simulink model "uz_pmsm_model_nonlinear"  (R2024b)
settings: Solver=FixedStepDiscrete  StartTime=0.0  StopTime=0.5  RelTol=1e-3
PreLoadFcn:
  | uz_pmsm_model_nonlinear_init_parameter
values from neighbouring files (symbols this model uses):
  ad1 = ad_1(1)    [LUT_approx_methode2a.m]    (also in LUT_approx_methode2a_clean.m = ad_self(1); LUT_approx_methode_2a_FEM.m; fitting_parameter.mat = 0.03048394862; fitting_parameter_48V_SynRM.mat = 0.0218446789236)
  ad2 = ad_1(2)    [LUT_approx_methode2a.m]    (also in LUT_approx_methode2a_clean.m = ad_self(2); LUT_approx_methode_2a_FEM.m; fitting_parameter.mat = 0.0402440194669; fitting_parameter_48V_SynRM.mat = 0.015691946268)
  ad3 = ad_1(3)    [LUT_approx_methode2a.m]    (also in LUT_approx_methode2a_clean.m = ad_self(3); LUT_approx_methode_2a_FEM.m; fitting_parameter.mat = -16.4812001193; fitting_parameter_48V_SynRM.mat = 2.77465564774)
  ad4 = ad_3_6(1)    [LUT_approx_methode2a.m]    (also in LUT_approx_methode2a_clean.m = ad_4_6(1); LUT_approx_methode_2a_FEM.m; fitting_parameter.mat = 1.2964378241; fitting_parameter_48V_SynRM.mat = 0.0214529395212)
  ad5 = ad_3_6(2)    [LUT_approx_methode2a.m]    (also in LUT_approx_methode2a_clean.m = ad_4_6(2); LUT_approx_methode_2a_FEM.m; fitting_parameter.mat = 0.000618316734858; fitting_parameter_48V_SynRM.mat = 0.0128514742508)
  ad6 = ad_3_6(3)    [LUT_approx_methode2a.m]    (also in LUT_approx_methode2a_clean.m = ad_4_6(3); LUT_approx_methode_2a_FEM.m; fitting_parameter.mat = -12.2755860444; fitting_parameter_48V_SynRM.mat = 2.54408267654)
  aq1 = aq_1(1)    [LUT_approx_methode2a.m]    (also in LUT_approx_methode2a_clean.m = aq_self(1); LUT_approx_methode_2a_FEM.m; fitting_parameter.mat = 0.0048166705291; fitting_parameter_48V_SynRM.mat = 0.00205546577039)
  aq2 = aq_1(2)    [LUT_approx_methode2a.m]    (also in LUT_approx_methode2a_clean.m = aq_self(2); LUT_approx_methode_2a_FEM.m; fitting_parameter.mat = 0.171595255564; fitting_parameter_48V_SynRM.mat = 0.0602932843871)
  aq3 = aq_1(3)    [LUT_approx_methode2a.m]    (also in LUT_approx_methode2a_clean.m = aq_self(3); LUT_approx_methode_2a_FEM.m; fitting_parameter.mat = 0.000926293864031; fitting_parameter_48V_SynRM.mat = 4.42738872822e-05)
  aq4 = aq_3_6(1)    [LUT_approx_methode2a.m]    (also in LUT_approx_methode2a_clean.m = aq_4_6(1); LUT_approx_methode_2a_FEM.m; fitting_parameter.mat = 0.00500187099075; fitting_parameter_48V_SynRM.mat = 0.000698420875152)
  aq5 = aq_3_6(2)    [LUT_approx_methode2a.m]    (also in LUT_approx_methode2a_clean.m = aq_4_6(2); LUT_approx_methode_2a_FEM.m; fitting_parameter.mat = 0.17052123489; fitting_parameter_48V_SynRM.mat = 0.0493122483219)
  aq6 = aq_3_6(3)    [LUT_approx_methode2a.m]    (also in LUT_approx_methode2a_clean.m = aq_4_6(3); LUT_approx_methode_2a_FEM.m; fitting_parameter.mat = 0.00091860845; fitting_parameter_48V_SynRM.mat = 4.14644316065e-05)
  Fid1_Giq1 = ((1/2).*(aq3-aq6).*((q_current_set).^2))+((aq1./aq2).*log(cosh(aq2.*q_current_set)))-((aq4/aq5).*log(cosh(aq5.*q_current_set)))    [LUT_approx_methode2a.m]    (also in LUT_approx_methode2a_clean.m; LUT_approx_methode_2a_FEM.m = (1/2).*(aq3-aq6).*((q_current_set).^2)+((aq1./aq2).*log(cosh; fitting_parameter.mat = -0.00135679401385; fitting_parameter_48V_SynRM.mat = 0.221350145237)
  Fid2_Giq2 = ((ad1./ad2).*(log(cosh(ad2.*(d_current_set-ad3))))) - ((ad4./ad5).*(log(cosh(ad5.*(d_current_set-ad6)))))    [LUT_approx_methode2a.m]    (also in LUT_approx_methode2a_clean.m; LUT_approx_methode_2a_FEM.m = ((ad1./ad2).*(log(cosh(ad2.*(d_current_set-ad3))))) - (((ad1; fitting_parameter.mat = 0.0788137932988; fitting_parameter_48V_SynRM.mat = 0.221214979406)
  friction_coefficient = 0.001    [uz_pmsm_model_init_parameter.m]    (also in uz_pmsm_model_init_parameter_clean.m)
  inertia = 0.000084    (= 8.4e-05)    [uz_pmsm_model_init_parameter.m]    (also in uz_pmsm_model_init_parameter_clean.m)
  k_i_d = R_1/(2*tau_sum)    (= 1875)    [uz_pmsm_model_init_parameter.m]    (also in uz_pmsm_model_init_parameter_clean.m)
  k_p_d = L_d/(2*tau_sum)    (= 2.8125)    [uz_pmsm_model_init_parameter.m]    (also in uz_pmsm_model_init_parameter_clean.m)
  k_p_q = L_q/(2*tau_sum)    (= 12.5)    [uz_pmsm_model_init_parameter.m]    (also in uz_pmsm_model_init_parameter_clean.m)
  L_d = 0.00045    [uz_pmsm_model_init_parameter.m]    (also in uz_pmsm_model_init_parameter_clean.m)
  L_q = 0.002    [uz_pmsm_model_init_parameter.m]    (also in uz_pmsm_model_init_parameter_clean.m)
  polepair = 4    [uz_pmsm_model_init_parameter.m]    (also in uz_pmsm_model_init_parameter_clean.m)
  psi_pm = 0.0194    [uz_pmsm_model_init_parameter.m]    (also in uz_pmsm_model_init_parameter_clean.m)
  R_1 = 0.3    [uz_pmsm_model_init_parameter.m]    (also in uz_pmsm_model_init_parameter_clean.m)
  setpoint_step = 4.0    (= 4)    [compare_simulation_to_measurement.m]    (also in export_csv.m = 10; iae_von_cil_measurements.m = 8; uz_pmsm_model_init_parameter.m = 10; uz_pmsm_model_init_parameter_clean.m = 10)
  simulate_mechanical = true    [compare_simulation_to_measurement.m]    (also in export_csv.m = false; uz_pmsm_model_init_parameter.m = false; uz_pmsm_model_init_parameter_clean.m = false)
  simulate_open_loop = true    [compare_simulation_to_measurement.m]    (also in export_csv.m; uz_pmsm_model_init_parameter.m = false; uz_pmsm_model_init_parameter_clean.m = false)
  static_friction_torque = 0.01    [uz_pmsm_model_init_parameter.m]    (also in uz_pmsm_model_init_parameter_clean.m)
  ts = logs{k}.Values    [export_csv.m]    (also in uz_pmsm_model_init_parameter.m = 2e-06; uz_pmsm_model_init_parameter_clean.m = 2e-06)
  ts_regler = 1/25e3    (= 4e-05)    [uz_pmsm_model_init_parameter.m]    (also in uz_pmsm_model_init_parameter_clean.m)
undefined symbols (not defined in the file or in its folder): simulate_nonlinear
libraries: slpidlib x2
settings Model: DataTypeOverride=Off  Creator=ts  LastModifiedBy=hufnagelde
settings SolverCC: AlgebraicLoopSolver=TrustRegion  AutoInsertRateTranBlk=on
settings DataIOCC: LimitDataPoints=on  SaveOutput=off  SaveTime=off
settings OptimizationCC: BlockReduction=off  ConditionallyExecuteInputs=off  DefaultParameterBehavior=Inlined  InheritOutputTypeSmallerThanSingle=on  LifeSpan=inf
settings DebuggingCC: AlgebraicLoopMsg=error  SingleTaskRateTransMsg=error  UnconnectedInputMsg=warning  UnconnectedOutputMsg=warning  UnconnectedLineMsg=warning  AllowSymbolicDim=off  StrictBusMsg=ErrorOnBusTreatedAsVector  SFUnexpectedBacktrackingDiag=warning  SFNoUnconditionalDefaultTransitionDiag=warning  SFExecutionAtInitializationDiag=none  ArithmeticOperatorsInVariantConditions=warning
settings HardwareCC: ProdBitPerPointer=32  ProdBitPerSizeT=32  ProdBitPerPtrDiffT=32  ProdLargestAtomicFloat=None  ProdIntDivRoundTo=Undefined  ProdEndianess=Unspecified  ProdWordSize=32  ProdHWDeviceType=ASIC/FPGA->ASIC/FPGA  ProdEqTarget=off
settings ModelReferenceCC: EnableRefExpFcnMdlSchedulingChecks=on
settings SFSimCC: SimUseLocalCustomCode=off  CustomCodeUndefinedFunction=UseInterfaceOnly
settings RTWCC: RTWUseLocalCustomCode=off  GPUComputeCapability=3.5  DLArmComputeVersion=19.05
settings CodeAppCC: StateflowObjectComments=on
settings GRTTargetCC: TargetLangStandard=C89/C90 (ANSI)
settings ConfigComp: CovScope=ReferencedModels  CovMetricSettings=dw  CovSaveCumulativeToWorkspaceVar=on  CovSaveSingleToWorkspaceVar=on  CovExternalEMLEnable=off  CovSFcnEnable=off

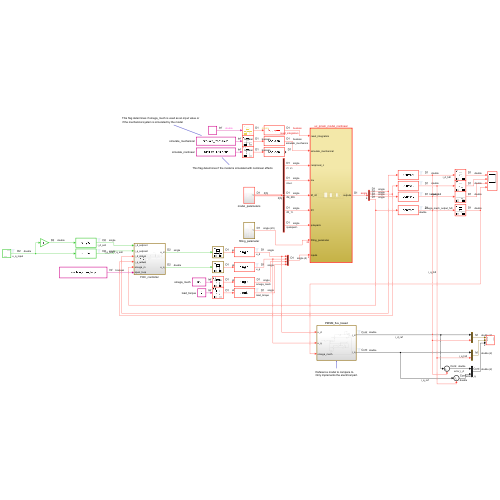
[thumbnail: Simulink's stored preview of the top-level diagram]
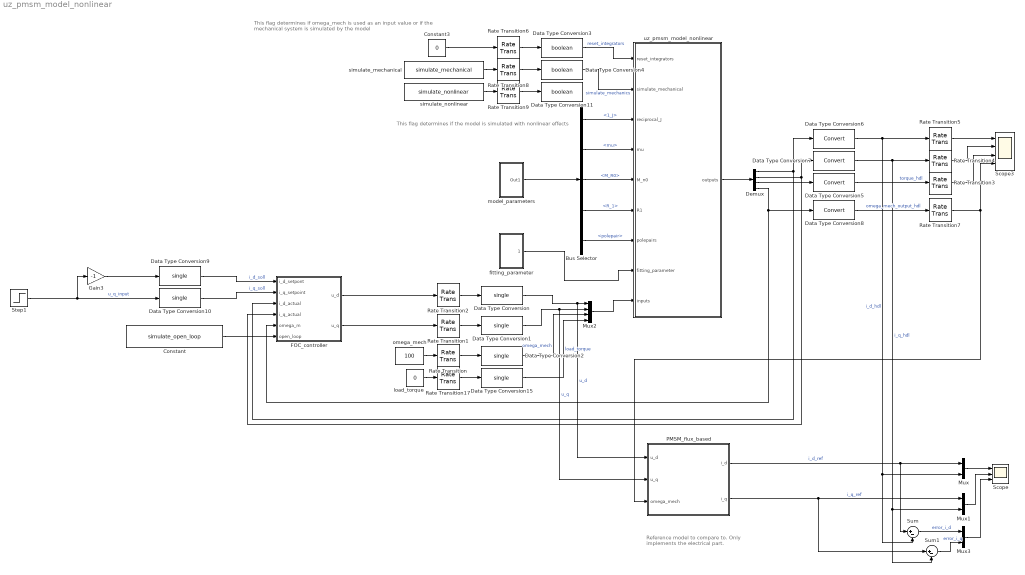
== system uz_pmsm_model_nonlinear ==
  note: This flag determines if the model is simulated with nonlinear effects
  note: Reference model to compare to.
      | Only implements the electrical part.
  note: This flag determines if omega_mech is used as an input value or
      | if the mechanical system is simulated by the model
  Bus Selector : BusSelector  OutputSignals=1_J,mu,M_R0,R_1,polepair
  Constant : Constant  Value=simulate_open_loop
  Constant3 : Constant  Value=0
  Data Type Conversion{,1..2,9..10,15} (6 alike) : DataTypeConversion  OutDataTypeStr=single  SaturateOnIntegerOverflow=off  RndMeth=Floor
  Data Type Conversion11 : DataTypeConversion  OutDataTypeStr=boolean  SaturateOnIntegerOverflow=off  RndMeth=Floor
  Data Type Conversion3 : DataTypeConversion  OutDataTypeStr=boolean  SaturateOnIntegerOverflow=off  RndMeth=Floor
  Data Type Conversion4 : DataTypeConversion  OutDataTypeStr=boolean  SaturateOnIntegerOverflow=off  RndMeth=Floor
  Data Type Conversion{5..8} (4 alike) : DataTypeConversion  SaturateOnIntegerOverflow=off  RndMeth=Floor
  Demux : Demux
  FOC_controller : Subsystem
  Gain3 : Gain  Gain=-1
  Mux : Mux  Inputs=2
  Mux1 : Mux  Inputs=2
  Mux2 : Mux
  Mux3 : Mux  Inputs=2
  PMSM_flux_based : Subsystem
  Rate Transition{,1..2,6,8..9,17} (7 alike) : RateTransition  OutPortSampleTime=ts
  Rate Transition{3..5,7} (4 alike) : RateTransition
  Scope : Scope  NumInputPorts=3
  Scope3 : Scope  NumInputPorts=4
  Step1 : Step  Time=0.2  After=setpoint_step  SampleTime=ts_regler
  Sum : Sum  Inputs=|+-
  Sum1 : Sum  Inputs=|+-
  fitting_parameter : Subsystem
  load_torque : Constant  Value=0
  model_parameters : Subsystem
  omega_mech : Constant  Value=100
  simulate_mechanical : Constant  Value=simulate_mechanical
  simulate_nonlinear : Constant  Value=simulate_nonlinear
  uz_pmsm_model_nonlinear : Subsystem  TreatAsAtomicUnit=on
  wires:
  Rate Transition/1 -> Data Type Conversion2/1
  Rate Transition1/1 -> Data Type Conversion1/1
  Rate Transition2/1 -> Data Type Conversion/1
  Data Type Conversion6/1 -> Mux/2, Sum/2, Rate Transition5/1  "i_d_hdl"
  Data Type Conversion7/1 -> Rate Transition4/1, Mux1/2, Sum1/2  "i_q_hdl"
  Data Type Conversion5/1 -> Rate Transition3/1  "torque_hdl"
  Rate Transition4/1 -> Scope3/2
  Rate Transition5/1 -> Scope3/1
  Rate Transition3/1 -> Scope3/3
  Rate Transition6/1 -> Data Type Conversion3/1
  Constant3/1 -> Rate Transition6/1
  Rate Transition8/1 -> Data Type Conversion4/1
  simulate_mechanical/1 -> Rate Transition8/1
  Data Type Conversion3/1 -> uz_pmsm_model_nonlinear/1(reset_integrators)  "reset_integrators"
  Data Type Conversion4/1 -> uz_pmsm_model_nonlinear/2(simulate_mechanical)  "simulate_mechanics"
  load_torque/1 -> Rate Transition17/1
  Rate Transition17/1 -> Data Type Conversion15/1
  Mux/1 -> Scope/1
  Mux1/1 -> Scope/2
  PMSM_flux_based/2(i_q) -> Mux1/1, Sum1/1  "i_q_ref"
  PMSM_flux_based/1(i_d) -> Mux/1, Sum/1  "i_d_ref"
  Data Type Conversion8/1 -> Rate Transition7/1  "omega_mech_output_hdl"
  Rate Transition7/1 -> PMSM_flux_based/3(omega_mech), Scope3/4
  Bus Selector/1 -> uz_pmsm_model_nonlinear/3(reciprocal_J)  "<1_J>"
  Bus Selector/2 -> uz_pmsm_model_nonlinear/4(mu)  "<mu>"
  Bus Selector/3 -> uz_pmsm_model_nonlinear/5(M_n0)  "<M_R0>"
  Bus Selector/4 -> uz_pmsm_model_nonlinear/6(R1)  "<R_1>"
  Bus Selector/5 -> uz_pmsm_model_nonlinear/7(polepairs)  "<polepair>"
  model_parameters/1(Out1) -> Bus Selector/1
  Sum/1 -> Mux3/1  "error_i_d"
  Sum1/1 -> Mux3/2  "error_i_q"
  Mux3/1 -> Scope/3
  Step1/1 -> Gain3/1, Data Type Conversion10/1  "u_q_input"
  Demux/3 -> Data Type Conversion5/1
  Gain3/1 -> Data Type Conversion9/1
  Demux/1 -> Data Type Conversion6/1, FOC_controller/3(i_d_actual)
  Demux/4 -> Data Type Conversion8/1, FOC_controller/5(omega_m)
  Demux/2 -> Data Type Conversion7/1, FOC_controller/4(i_q_actual)
  Data Type Conversion/1 -> PMSM_flux_based/1(u_d), Mux2/1  "u_d"
  Data Type Conversion1/1 -> PMSM_flux_based/2(u_q), Mux2/2  "u_q"
  Data Type Conversion15/1 -> Mux2/4  "load_torque"
  Data Type Conversion2/1 -> Mux2/3  "omega_mech"
  Mux2/1 -> uz_pmsm_model_nonlinear/9(inputs)
  uz_pmsm_model_nonlinear/1(outputs) -> Demux/1
  Data Type Conversion9/1 -> FOC_controller/1(i_d_setpont)  "i_d_soll"
  Data Type Conversion10/1 -> FOC_controller/2(i_q_setpoint)  "i_q_soll"
  FOC_controller/1(u_d) -> Rate Transition2/1
  FOC_controller/2(u_q) -> Rate Transition1/1
  omega_mech/1 -> Rate Transition/1
  Constant/1 -> FOC_controller/6(open_loop)
  simulate_nonlinear/1 -> Rate Transition9/1
  Rate Transition9/1 -> Data Type Conversion11/1
  fitting_parameter/1(1) -> uz_pmsm_model_nonlinear/8(fitting_parameter)

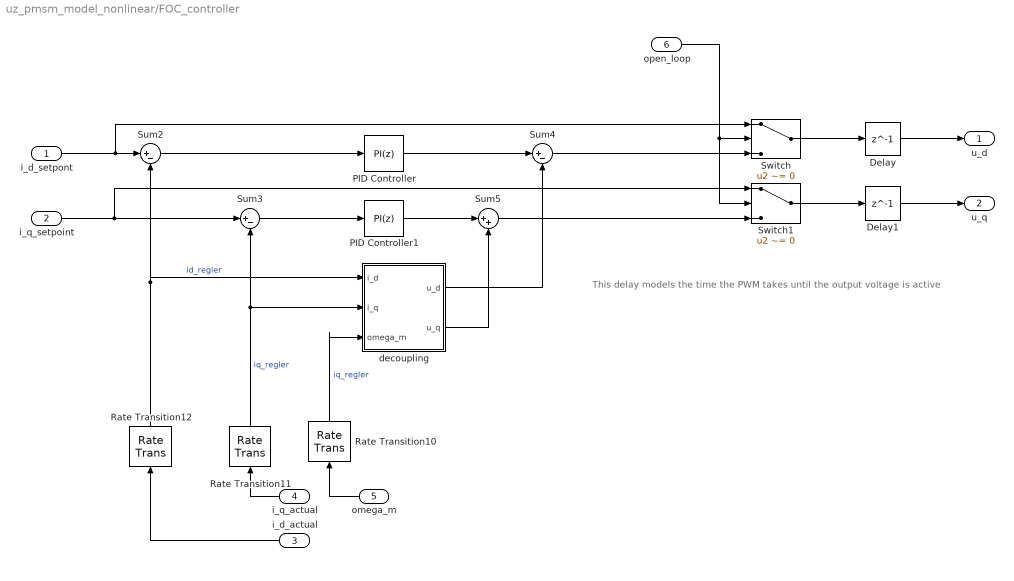
== system uz_pmsm_model_nonlinear/FOC_controller ==
  note: This delay models the time the PWM takes until the output voltage is active
  i_d_setpont : Inport
  i_q_setpoint : Inport  Port=2
  i_d_actual : Inport  Port=3
  i_q_actual : Inport  Port=4
  omega_m : Inport  Port=5
  open_loop : Inport  Port=6
  Delay : Delay  DelayLength=1
  Delay1 : Delay  DelayLength=1
  PID Controller : slpidlib/PID Controller  Controller=PI  Form=Parallel  TimeDomain=Discrete-time  UseExternalTs=off  SampleTime=-1  IntegratorMethod=Forward Euler  FilterMethod=Forward Euler  ControllerParametersSource=internal  P=k_p_d  I=k_i_d  UseKiTs=off  D=0  UseExternalDerivativeSource=off  N=100  UseFilter=on  TunerSelectOption=Transfer Function Based (PID Tuner App)  InitialConditionSource=internal  InitialConditionForIntegrator=0  InitialConditionForFilter=0  DifferentiatorICPrevScaledInput=0  ExternalReset=none  TrackingMode=off  Kt=1  LimitOutput=off  SatLimitsSource=internal  UpperSaturationLimit=inf  LowerSaturationLimit=-inf  LinearizeAsGain=on  AntiWindupMode=none  Kb=1  LimitIntegrator=off  UpperIntegratorSaturationLimit=inf  LowerIntegratorSaturationLimit=-inf  POutMin=[]  POutMax=[]  IOutMin=[]  IOutMax=[]  DOutMin=[]  DOutMax=[]  NOutMin=[]  NOutMax=[]  SumOutMin=[]  SumOutMax=[]  SaturationOutMin=[]  SaturationOutMax=[]  PParamMin=[]  PParamMax=[]  IParamMin=[]  IParamMax=[]  DParamMin=[]  DParamMax=[]  NParamMin=[]  NParamMax=[]  KbParamMin=[]  KbParamMax=[]  KtParamMin=[]  KtParamMax=[]  KbOutMin=[]  KbOutMax=[]  KtOutMin=[]  KtOutMax=[]  IntegratorOutMin=[]  IntegratorOutMax=[]  FilterOutMin=[]  FilterOutMax=[]  SumI1OutMin=[]  SumI1OutMax=[]  SumI2OutMin=[]  SumI2OutMax=[]  SumI3OutMin=[]  SumI3OutMax=[]  SumI4OutMin=[]  SumI4OutMax=[]  SumDOutMin=[]  SumDOutMax=[]  DifferentiatorOutMin=[]  DifferentiatorOutMax=[]  FilterDiffOutCoefMin=[]  FilterDiffOutCoefMax=[]  ReciprocalOutMin=[]  ReciprocalOutMax=[]  SumDenOutMin=[]  SumDenOutMax=[]  SumNumOutMin=[]  SumNumOutMax=[]  DivideOutMin=[]  DivideOutMax=[]  UdiffTsProdOutMin=[]  UdiffTsProdOutMax=[]  NTsProdOutMin=[]  NTsProdOutMax=[]  UintegralTsProdOutMin=[]  UintegralTsProdOutMax=[]  UngainTsProdOutMin=[]  UngainTsProdOutMax=[]  ClampingZeroOutDataTypeStr=Inherit: Inherit via back propagation  ClampingZeroOutMin=[]  ClampingZeroOutMax=[]  FilterDenConstantOutDataTypeStr=Inherit: Inherit via back propagation  FilterDenConstantOutMin=[]  FilterDenConstantOutMax=[]  PCopyOutDataTypeStr=Inherit: Inherit via back propagation  PCopyOutMin=[]  PCopyOutMax=[]  NCopyOutDataTypeStr=Inherit: Inherit via back propagation  NCopyOutMin=[]  NCopyOutMax=[]  IntegratorContinuousStateAttributes=''  IntegratorStateMustResolveToSignalObject=off  IntegratorRTWStateStorageClass=Auto  FilterContinuousStateAttributes=''  FilterStateMustResolveToSignalObject=off  FilterRTWStateStorageClass=Auto  ParallelPVariant=InternalParameters  IdealPVariant=Disabled  IVariant=InternalParameters  DVariant=Disabled  IntegratorVariant=Discrete  SatVariant=Disabled  AWVariant=Passthrough  PCopyVariant=Disabled  TRVariant=Disabled  FdbkBlocksVariant=Forward  IdealPFdbkVariant=Disabled  SatFdbkVariant=Disabled  DerivativeFilterVariant=Disabled  NVariant=Disabled  NCopyVariant=Disabled_SignalSpec  FilterICVariant=Disabled  IntegratorICVariant=InternalICs  ExternalResetVariant=Disabled  TRSumVariant=Passthrough  SumFdbkVariant=Disabled  SumVariant=Sum_PI  TsampFilterVariant=InternalTs  TsampNgainVariant=Passthrough  TsampIntegralVariant=Disabled_SignalSpec  ExternalSaturationOutDataTypeStr=Inherit: Same as second input  DerivativeSourceVariant=Disabled  PreIntVariant=InternalPreInt
  PID Controller1 : slpidlib/PID Controller  Controller=PI  Form=Parallel  TimeDomain=Discrete-time  UseExternalTs=off  SampleTime=-1  IntegratorMethod=Forward Euler  FilterMethod=Forward Euler  ControllerParametersSource=internal  P=k_p_q  I=k_i_d  UseKiTs=off  D=0  UseExternalDerivativeSource=off  N=100  UseFilter=on  TunerSelectOption=Transfer Function Based (PID Tuner App)  InitialConditionSource=internal  InitialConditionForIntegrator=0  InitialConditionForFilter=0  DifferentiatorICPrevScaledInput=0  ExternalReset=none  TrackingMode=off  Kt=1  LimitOutput=off  SatLimitsSource=internal  UpperSaturationLimit=inf  LowerSaturationLimit=-inf  LinearizeAsGain=on  AntiWindupMode=none  Kb=1  LimitIntegrator=off  UpperIntegratorSaturationLimit=inf  LowerIntegratorSaturationLimit=-inf  POutMin=[]  POutMax=[]  IOutMin=[]  IOutMax=[]  DOutMin=[]  DOutMax=[]  NOutMin=[]  NOutMax=[]  SumOutMin=[]  SumOutMax=[]  SaturationOutMin=[]  SaturationOutMax=[]  PParamMin=[]  PParamMax=[]  IParamMin=[]  IParamMax=[]  DParamMin=[]  DParamMax=[]  NParamMin=[]  NParamMax=[]  KbParamMin=[]  KbParamMax=[]  KtParamMin=[]  KtParamMax=[]  KbOutMin=[]  KbOutMax=[]  KtOutMin=[]  KtOutMax=[]  IntegratorOutMin=[]  IntegratorOutMax=[]  FilterOutMin=[]  FilterOutMax=[]  SumI1OutMin=[]  SumI1OutMax=[]  SumI2OutMin=[]  SumI2OutMax=[]  SumI3OutMin=[]  SumI3OutMax=[]  SumI4OutMin=[]  SumI4OutMax=[]  SumDOutMin=[]  SumDOutMax=[]  DifferentiatorOutMin=[]  DifferentiatorOutMax=[]  FilterDiffOutCoefMin=[]  FilterDiffOutCoefMax=[]  ReciprocalOutMin=[]  ReciprocalOutMax=[]  SumDenOutMin=[]  SumDenOutMax=[]  SumNumOutMin=[]  SumNumOutMax=[]  DivideOutMin=[]  DivideOutMax=[]  UdiffTsProdOutMin=[]  UdiffTsProdOutMax=[]  NTsProdOutMin=[]  NTsProdOutMax=[]  UintegralTsProdOutMin=[]  UintegralTsProdOutMax=[]  UngainTsProdOutMin=[]  UngainTsProdOutMax=[]  ClampingZeroOutDataTypeStr=Inherit: Inherit via back propagation  ClampingZeroOutMin=[]  ClampingZeroOutMax=[]  FilterDenConstantOutDataTypeStr=Inherit: Inherit via back propagation  FilterDenConstantOutMin=[]  FilterDenConstantOutMax=[]  PCopyOutDataTypeStr=Inherit: Inherit via back propagation  PCopyOutMin=[]  PCopyOutMax=[]  NCopyOutDataTypeStr=Inherit: Inherit via back propagation  NCopyOutMin=[]  NCopyOutMax=[]  IntegratorContinuousStateAttributes=''  IntegratorStateMustResolveToSignalObject=off  IntegratorRTWStateStorageClass=Auto  FilterContinuousStateAttributes=''  FilterStateMustResolveToSignalObject=off  FilterRTWStateStorageClass=Auto  ParallelPVariant=InternalParameters  IdealPVariant=Disabled  IVariant=InternalParameters  DVariant=Disabled  IntegratorVariant=Discrete  SatVariant=Disabled  AWVariant=Passthrough  PCopyVariant=Disabled  TRVariant=Disabled  FdbkBlocksVariant=Forward  IdealPFdbkVariant=Disabled  SatFdbkVariant=Disabled  DerivativeFilterVariant=Disabled  NVariant=Disabled  NCopyVariant=Disabled_SignalSpec  FilterICVariant=Disabled  IntegratorICVariant=InternalICs  ExternalResetVariant=Disabled  TRSumVariant=Passthrough  SumFdbkVariant=Disabled  SumVariant=Sum_PI  TsampFilterVariant=InternalTs  TsampNgainVariant=Passthrough  TsampIntegralVariant=Disabled_SignalSpec  ExternalSaturationOutDataTypeStr=Inherit: Same as second input  DerivativeSourceVariant=Disabled  PreIntVariant=InternalPreInt
  Rate Transition10 : RateTransition  OutPortSampleTime=ts_regler
  Rate Transition11 : RateTransition  OutPortSampleTime=ts_regler
  Rate Transition12 : RateTransition  OutPortSampleTime=ts_regler
  Sum2 : Sum  Inputs=|+-
  Sum3 : Sum  Inputs=|+-
  Sum4 : Sum  Inputs=|+-
  Sum5 : Sum  Inputs=|++
  Switch : Switch  Criteria=u2 ~= 0  SaturateOnIntegerOverflow=off  InputSameDT=off
  Switch1 : Switch  Criteria=u2 ~= 0  SaturateOnIntegerOverflow=off  InputSameDT=off
  decoupling : Subsystem
  u_d : Outport
  u_q : Outport  Port=2
  wires:
  PID Controller/1 -> Sum4/1
  PID Controller1/1 -> Sum5/1
  Sum4/1 -> Switch/3
  i_d_actual/1 -> Rate Transition12/1
  i_d_setpont/1 -> Switch/1, Sum2/1
  Sum2/1 -> PID Controller/1
  Sum5/1 -> Switch1/3
  omega_m/1 -> Rate Transition10/1
  Sum3/1 -> PID Controller1/1
  i_q_actual/1 -> Rate Transition11/1
  Rate Transition12/1 -> decoupling/1(i_d), Sum2/2  "id_regler"
  Rate Transition11/1 -> decoupling/2(i_q), Sum3/2  "iq_regler"
  i_q_setpoint/1 -> Switch1/1, Sum3/1
  open_loop/1 -> Switch1/2, Switch/2
  Rate Transition10/1 -> decoupling/3(omega_m)  "iq_regler"
  decoupling/1(u_d) -> Sum4/2
  decoupling/2(u_q) -> Sum5/2
  Switch/1 -> Delay/1
  Switch1/1 -> Delay1/1
  Delay/1 -> u_d/1
  Delay1/1 -> u_q/1

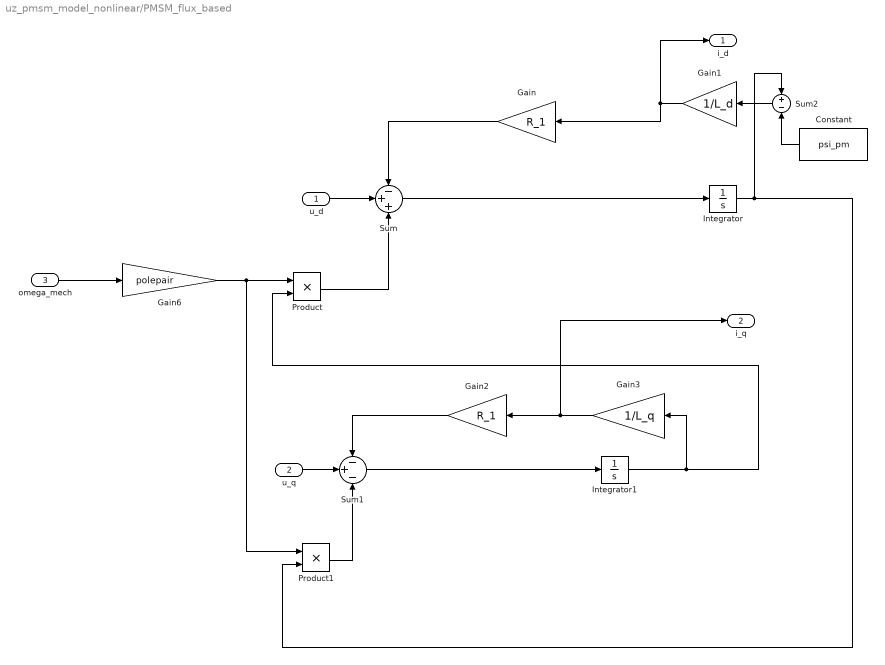
== system uz_pmsm_model_nonlinear/PMSM_flux_based ==
  u_d : Inport
  u_q : Inport  Port=2
  omega_mech : Inport  Port=3
  Constant : Constant  Value=psi_pm
  Gain : Gain  Gain=R_1
  Gain1 : Gain  Gain=1/L_d
  Gain2 : Gain  Gain=R_1
  Gain3 : Gain  Gain=1/L_q
  Gain6 : Gain  Gain=polepair
  Integrator : Integrator
  Integrator1 : Integrator
  Product : Product
  Product1 : Product
  Sum : Sum  Inputs=-++
  Sum1 : Sum  Inputs=-+-
  Sum2 : Sum  Inputs=+-
  i_d : Outport
  i_q : Outport  Port=2
  wires:
  u_d/1 -> Sum/2
  u_q/1 -> Sum1/2
  Sum/1 -> Integrator/1
  Gain/1 -> Sum/1
  Integrator/1 -> Product1/2, Sum2/1
  Constant/1 -> Sum2/2
  Sum2/1 -> Gain1/1
  Gain1/1 -> Gain/1, i_d/1
  Gain6/1 -> Product1/1, Product/1
  Product/1 -> Sum/3
  Integrator1/1 -> Gain3/1, Product/2
  Product1/1 -> Sum1/3
  Sum1/1 -> Integrator1/1
  Gain2/1 -> Sum1/1
  Gain3/1 -> i_q/1, Gain2/1
  omega_mech/1 -> Gain6/1

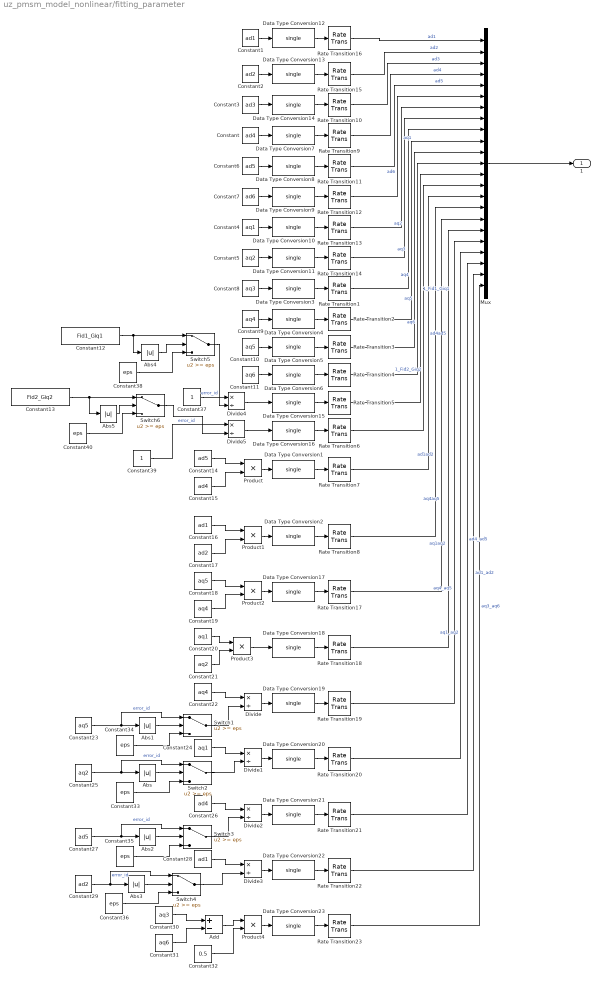
== system uz_pmsm_model_nonlinear/fitting_parameter ==
  Abs{,1..5} (6 alike) : Abs  SaturateOnIntegerOverflow=off
  Add : Sum  Inputs=+-
  Constant : Constant  Value=ad4
  Constant1 : Constant  Value=ad1
  Constant10 : Constant  Value=aq5
  Constant11 : Constant  Value=aq6
  Constant12 : Constant  Value=Fid1_Giq1
  Constant13 : Constant  Value=Fid2_Giq2
  Constant14 : Constant  Value=ad5
  Constant15 : Constant  Value=ad4
  Constant16 : Constant  Value=ad1
  Constant17 : Constant  Value=ad2
  Constant18 : Constant  Value=aq5
  Constant19 : Constant  Value=aq4
  Constant2 : Constant  Value=ad2
  Constant20 : Constant  Value=aq1
  Constant21 : Constant  Value=aq2
  Constant22 : Constant  Value=aq4
  Constant23 : Constant  Value=aq5
  Constant24 : Constant  Value=aq1
  Constant25 : Constant  Value=aq2
  Constant26 : Constant  Value=ad4
  Constant27 : Constant  Value=ad5
  Constant28 : Constant  Value=ad1
  Constant29 : Constant  Value=ad2
  Constant3 : Constant  Value=ad3
  Constant30 : Constant  Value=aq3
  Constant31 : Constant  Value=aq6
  Constant32 : Constant  Value=0.5  OutDataTypeStr=double  SampleTime=-1
  Constant{33..36,38,40} (6 alike) : Constant  Value=eps  SampleTime=ts_regler
  Constant37 : Constant
  Constant39 : Constant
  Constant4 : Constant  Value=aq1
  Constant5 : Constant  Value=aq2
  Constant6 : Constant  Value=ad5
  Constant7 : Constant  Value=ad6
  Constant8 : Constant  Value=aq3
  Constant9 : Constant  Value=aq4
  Data Type Conversion{1..23} (23 alike) : DataTypeConversion  OutDataTypeStr=single  SaturateOnIntegerOverflow=off  RndMeth=Floor
  Divide{,1..5} (6 alike) : Product  Inputs=*/
  Mux : Mux  Inputs=23
  Product{,1..4} (5 alike) : Product
  Rate Transition{1..23} (23 alike) : RateTransition  OutPortSampleTime=ts
  Switch{1..6} (6 alike) : Switch  Threshold=eps  SaturateOnIntegerOverflow=off  InputSameDT=off
  1 : Outport
  wires:
  Constant1/1 -> Data Type Conversion12/1
  Constant/1 -> Data Type Conversion7/1
  Rate Transition10/1 -> Mux/3  "ad3"
  Rate Transition14/1 -> Mux/8  "aq2"
  Constant3/1 -> Data Type Conversion14/1
  Rate Transition12/1 -> Mux/6  "ad6"
  Rate Transition16/1 -> Mux/1  "ad1"
  Rate Transition13/1 -> Mux/7  "aq1"
  Constant5/1 -> Data Type Conversion11/1
  Constant7/1 -> Data Type Conversion9/1
  Rate Transition15/1 -> Mux/2  "ad2"
  Rate Transition9/1 -> Mux/4  "ad4"
  Constant6/1 -> Data Type Conversion8/1
  Constant4/1 -> Data Type Conversion10/1
  Rate Transition11/1 -> Mux/5  "ad5"
  Constant2/1 -> Data Type Conversion13/1
  Rate Transition1/1 -> Mux/9  "aq3"
  Constant8/1 -> Data Type Conversion3/1
  Rate Transition2/1 -> Mux/10  "aq4"
  Constant9/1 -> Data Type Conversion4/1
  Rate Transition3/1 -> Mux/11  "aq5"
  Constant10/1 -> Data Type Conversion5/1
  Rate Transition4/1 -> Mux/12  "aq6"
  Constant11/1 -> Data Type Conversion6/1
  Rate Transition5/1 -> Mux/13  "1_Fid1_Giq1"
  Rate Transition6/1 -> Mux/14  "1_Fid2_Giq2"
  Data Type Conversion11/1 -> Rate Transition14/1
  Data Type Conversion10/1 -> Rate Transition13/1
  Data Type Conversion9/1 -> Rate Transition12/1
  Data Type Conversion12/1 -> Rate Transition16/1
  Data Type Conversion13/1 -> Rate Transition15/1
  Data Type Conversion14/1 -> Rate Transition10/1
  Data Type Conversion7/1 -> Rate Transition9/1
  Data Type Conversion8/1 -> Rate Transition11/1
  Data Type Conversion3/1 -> Rate Transition1/1
  Data Type Conversion4/1 -> Rate Transition2/1
  Data Type Conversion5/1 -> Rate Transition3/1
  Data Type Conversion6/1 -> Rate Transition4/1
  Data Type Conversion15/1 -> Rate Transition5/1
  Data Type Conversion16/1 -> Rate Transition6/1
  Constant14/1 -> Product/1
  Constant15/1 -> Product/2
  Product/1 -> Data Type Conversion1/1
  Data Type Conversion1/1 -> Rate Transition7/1
  Rate Transition7/1 -> Mux/15  "ad4ad5"
  Rate Transition8/1 -> Mux/16  "ad1ad2"
  Constant16/1 -> Product1/1
  Constant17/1 -> Product1/2
  Data Type Conversion2/1 -> Rate Transition8/1
  Product1/1 -> Data Type Conversion2/1
  Constant18/1 -> Product2/1
  Constant19/1 -> Product2/2
  Data Type Conversion17/1 -> Rate Transition17/1
  Product2/1 -> Data Type Conversion17/1
  Rate Transition18/1 -> Mux/18  "aq1aq2"
  Product3/1 -> Data Type Conversion18/1
  Data Type Conversion18/1 -> Rate Transition18/1
  Constant21/1 -> Product3/2
  Constant20/1 -> Product3/1
  Rate Transition17/1 -> Mux/17  "aq4aq5"
  Divide/1 -> Data Type Conversion19/1
  Data Type Conversion19/1 -> Rate Transition19/1
  Constant22/1 -> Divide/1
  Rate Transition19/1 -> Mux/19  "aq4_aq5"
  Constant24/1 -> Divide1/1
  Rate Transition20/1 -> Mux/20  "aq1_aq2"
  Divide1/1 -> Data Type Conversion20/1
  Data Type Conversion20/1 -> Rate Transition20/1
  Data Type Conversion21/1 -> Rate Transition21/1
  Divide2/1 -> Data Type Conversion21/1
  Rate Transition21/1 -> Mux/21  "ad4_ad5"
  Constant26/1 -> Divide2/1
  Constant28/1 -> Divide3/1
  Rate Transition22/1 -> Mux/22  "ad1_ad2"
  Divide3/1 -> Data Type Conversion22/1
  Data Type Conversion22/1 -> Rate Transition22/1
  Data Type Conversion23/1 -> Rate Transition23/1
  Constant30/1 -> Add/1
  Constant31/1 -> Add/2
  Rate Transition23/1 -> Mux/23  "aq3_aq6"
  Product4/1 -> Data Type Conversion23/1
  Constant32/1 -> Product4/2
  Add/1 -> Product4/1
  Mux/1 -> 1/1
  Constant25/1 -> Switch2/1, Abs/1  "error_id"
  Switch2/1 -> Divide1/2
  Abs/1 -> Switch2/2
  Constant33/1 -> Switch2/3
  Constant23/1 -> Switch1/1, Abs1/1  "error_id"
  Switch1/1 -> Divide/2
  Abs1/1 -> Switch1/2
  Constant34/1 -> Switch1/3
  Constant27/1 -> Switch3/1, Abs2/1  "error_id"
  Switch3/1 -> Divide2/2
  Abs2/1 -> Switch3/2
  Constant35/1 -> Switch3/3
  Constant29/1 -> Switch4/1, Abs3/1  "error_id"
  Switch4/1 -> Divide3/2
  Abs3/1 -> Switch4/2
  Constant36/1 -> Switch4/3
  Abs4/1 -> Switch5/2
  Constant38/1 -> Switch5/3
  Divide4/1 -> Data Type Conversion15/1
  Switch5/1 -> Divide4/2
  Constant12/1 -> Switch5/1, Abs4/1
  Constant37/1 -> Divide4/1  "error_id"
  Constant39/1 -> Divide5/1  "error_id"
  Constant13/1 -> Abs5/1, Switch6/1
  Constant40/1 -> Switch6/3
  Abs5/1 -> Switch6/2
  Divide5/1 -> Data Type Conversion16/1
  Switch6/1 -> Divide5/2

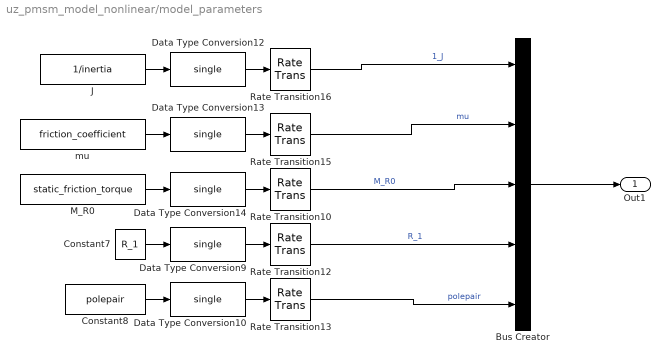
== system uz_pmsm_model_nonlinear/model_parameters ==
  Bus Creator : BusCreator  Inputs=5
  Constant7 : Constant  Value=R_1
  Constant8 : Constant  Value=polepair
  Data Type Conversion{9..10,12..14} (5 alike) : DataTypeConversion  OutDataTypeStr=single  SaturateOnIntegerOverflow=off  RndMeth=Floor
  J : Constant  Value=1/inertia
  M_R0 : Constant  Value=static_friction_torque
  Rate Transition{10,12..13,15..16} (5 alike) : RateTransition  OutPortSampleTime=ts
  mu : Constant  Value=friction_coefficient
  Out1 : Outport
  wires:
  Data Type Conversion12/1 -> Rate Transition16/1
  Rate Transition10/1 -> Bus Creator/3  "M_R0"
  Data Type Conversion14/1 -> Rate Transition10/1
  Rate Transition12/1 -> Bus Creator/4  "R_1"
  Rate Transition16/1 -> Bus Creator/1  "1_J"
  Rate Transition13/1 -> Bus Creator/5  "polepair"
  Bus Creator/1 -> Out1/1
  Constant8/1 -> Data Type Conversion10/1
  Data Type Conversion9/1 -> Rate Transition12/1
  Rate Transition15/1 -> Bus Creator/2  "mu"
  J/1 -> Data Type Conversion12/1
  Data Type Conversion10/1 -> Rate Transition13/1
  mu/1 -> Data Type Conversion13/1
  M_R0/1 -> Data Type Conversion14/1
  Data Type Conversion13/1 -> Rate Transition15/1
  Constant7/1 -> Data Type Conversion9/1

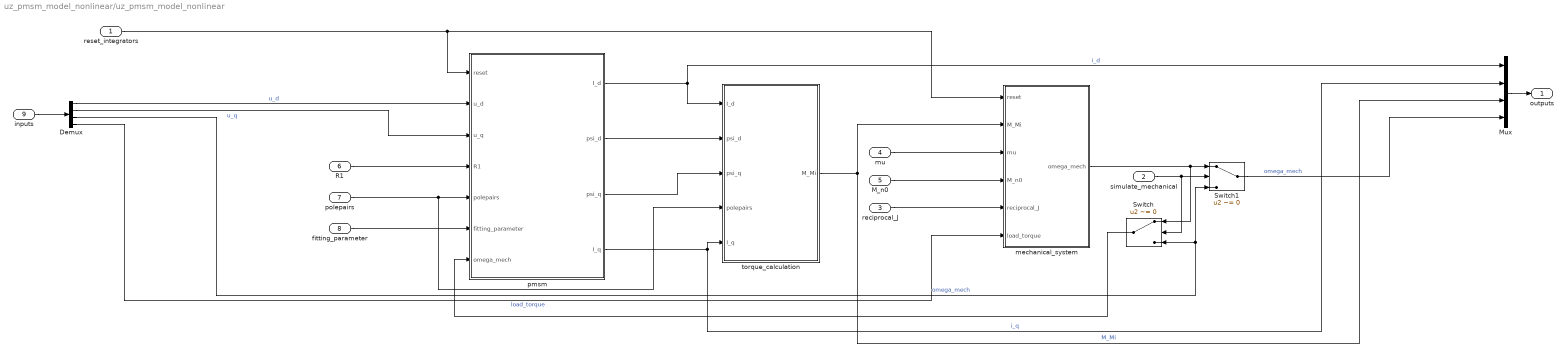
== system uz_pmsm_model_nonlinear/uz_pmsm_model_nonlinear ==
  reset_integrators : Inport
  simulate_mechanical : Inport  Port=2
  reciprocal_J : Inport  Port=3
  mu : Inport  Port=4
  M_n0 : Inport  Port=5
  R1 : Inport  Port=6
  polepairs : Inport  Port=7
  fitting_parameter : Inport  Port=8
  inputs : Inport  Port=9
  Demux : Demux
  Mux : Mux
  Switch : Switch  Criteria=u2 ~= 0  SaturateOnIntegerOverflow=off  InputSameDT=off
  Switch1 : Switch  Criteria=u2 ~= 0  SaturateOnIntegerOverflow=off  InputSameDT=off
  mechanical_system : Subsystem
  pmsm : Subsystem
  torque_calculation : Subsystem
  outputs : Outport
  wires:
  reset_integrators/1 -> pmsm/1(reset), mechanical_system/1(reset)
  Demux/3 -> Switch1/3, Switch/3  "omega_mech"
  Switch/1 -> pmsm/7(omega_mech)
  pmsm/2(psi_d) -> torque_calculation/2(psi_d)
  Demux/4 -> mechanical_system/6(load_torque)  "load_torque"
  R1/1 -> pmsm/4(R1)
  pmsm/3(psi_q) -> torque_calculation/3(psi_q)
  polepairs/1 -> torque_calculation/4(polepairs), pmsm/5(polepairs)
  Demux/1 -> pmsm/2(u_d)  "u_d"
  mu/1 -> mechanical_system/3(mu)
  simulate_mechanical/1 -> Switch1/2, Switch/2
  reciprocal_J/1 -> mechanical_system/5(reciprocal_J)
  M_n0/1 -> mechanical_system/4(M_n0)
  Demux/2 -> pmsm/3(u_q)  "u_q"
  mechanical_system/1(omega_mech) -> Switch/1, Switch1/1
  pmsm/4(I_q) -> Mux/2, torque_calculation/5(I_q)  "i_q"
  pmsm/1(I_d) -> torque_calculation/1(I_d), Mux/1  "i_d"
  Switch1/1 -> Mux/4  "omega_mech"
  torque_calculation/1(M_Mi) -> mechanical_system/2(M_Mi), Mux/3  "M_Mi"
  inputs/1 -> Demux/1
  Mux/1 -> outputs/1
  fitting_parameter/1 -> pmsm/6(fitting_parameter)

== system uz_pmsm_model_nonlinear/FOC_controller/decoupling ==
  i_d : Inport
  i_q : Inport  Port=2
  omega_m : Inport  Port=3
  Constant1 : Constant  Value=psi_pm  SampleTime=-1
  Gain : Gain  Gain=L_q
  Gain1 : Gain  Gain=L_d
  Gain2 : Gain  Gain=polepair
  Product : Product
  Product1 : Product
  Sum6 : Sum  Inputs=|++
  u_d : Outport
  u_q : Outport  Port=2
  wires:
  Gain/1 -> Product/1
  Gain2/1 -> Product1/2, Product/2
  Product1/1 -> u_q/1
  i_d/1 -> Gain1/1
  Product/1 -> u_d/1
  Gain1/1 -> Sum6/1
  i_q/1 -> Gain/1
  Constant1/1 -> Sum6/2
  Sum6/1 -> Product1/1
  omega_m/1 -> Gain2/1

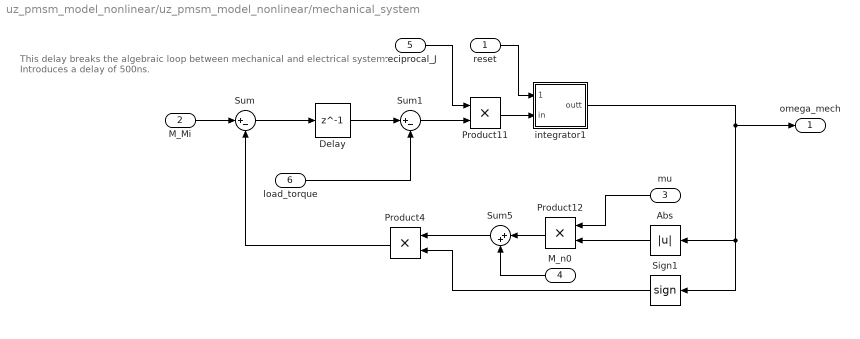
== system uz_pmsm_model_nonlinear/uz_pmsm_model_nonlinear/mechanical_system ==
  note: This delay breaks the algebraic loop between mechanical and electrical system.
      | Introduces a delay of 500ns.
  reset : Inport
  M_Mi : Inport  Port=2
  mu : Inport  Port=3
  M_n0 : Inport  Port=4
  reciprocal_J : Inport  Port=5
  load_torque : Inport  Port=6
  Abs : Abs  SaturateOnIntegerOverflow=off
  Delay : Delay  DelayLength=1
  Product11 : Product
  Product12 : Product
  Product4 : Product
  Sign1 : Signum
  Sum : Sum  Inputs=|+-
  Sum1 : Sum  Inputs=|+-
  Sum5 : Sum  Inputs=|++
  integrator1 : Subsystem
  omega_mech : Outport
  wires:
  Product11/1 -> integrator1/2(in)
  Sum5/1 -> Product4/1
  Sign1/1 -> Product4/2
  integrator1/1(outt) -> Sign1/1, Abs/1, omega_mech/1
  Abs/1 -> Product12/2
  reset/1 -> integrator1/1(reset)
  Product12/1 -> Sum5/1
  mu/1 -> Product12/1
  M_n0/1 -> Sum5/2
  reciprocal_J/1 -> Product11/1
  M_Mi/1 -> Sum/1
  Sum1/1 -> Product11/2
  load_torque/1 -> Sum1/2
  Sum/1 -> Delay/1
  Product4/1 -> Sum/2
  Delay/1 -> Sum1/1

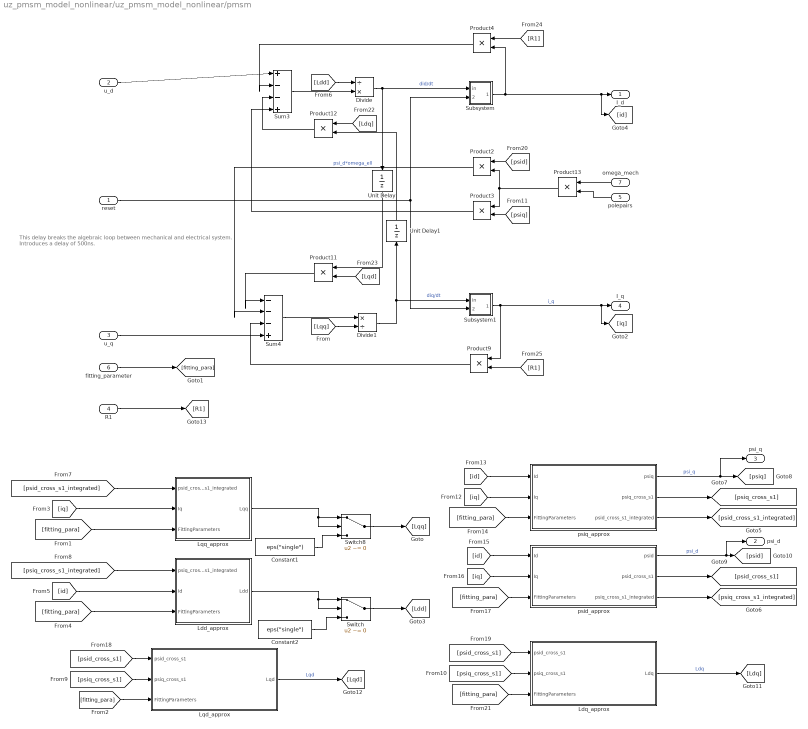
== system uz_pmsm_model_nonlinear/uz_pmsm_model_nonlinear/pmsm ==
  note: This delay breaks the algebraic loop between mechanical and electrical system.
      | Introduces a delay of 500ns.
  reset : Inport
  u_d : Inport  Port=2
  u_q : Inport  Port=3
  R1 : Inport  Port=4
  polepairs : Inport  Port=5
  fitting_parameter : Inport  Port=6
  omega_mech : Inport  Port=7
  Constant1 : Constant  Value="eps(\"single\")"  OutDataTypeStr=single  SampleTime=ts
  Constant2 : Constant  Value="eps(\"single\")"  OutDataTypeStr=single  SampleTime=ts
  Divide : Product  Inputs=/*  OutDataTypeStr=Inherit: Same as first input
  Divide1 : Product  Inputs=*/  OutDataTypeStr=Inherit: Same as first input
  Ldd_approx : Subsystem
  Ldq_approx : Subsystem
  Lqd_approx : Subsystem
  Lqq_approx : Subsystem
  Product11 : Product
  Product{2,4,9,12..13} (5 alike) : Product  OutDataTypeStr=Inherit: Same as first input
  Product3 : Product
  Subsystem : Subsystem
  Subsystem1 : Subsystem
  Sum3 : Sum  Inputs=|+--+  OutDataTypeStr=Inherit: Same as first input
  Sum4 : Sum  Inputs=|---+
  Switch : Switch  Criteria=u2 ~= 0  Threshold="eps(\"single\")"  SaturateOnIntegerOverflow=off  InputSameDT=off
  Switch8 : Switch  Criteria=u2 ~= 0  SaturateOnIntegerOverflow=off  InputSameDT=off
  Unit Delay : UnitDelay  SampleTime=-1  HasFrameUpgradeWarning=on
  Unit Delay1 : UnitDelay  SampleTime=-1  HasFrameUpgradeWarning=on
  psid_approx : Subsystem
  psiq_approx : Subsystem
  I_d : Outport
  psi_d : Outport  Port=2
  psi_q : Outport  Port=3
  I_q : Outport  Port=4
  wires:
  Sum4/1 -> Divide1/1
  u_q/1 -> Sum4/4
  Divide1/1 -> Unit Delay1/1, Subsystem1/1(in)  "diq/dt"
  polepairs/1 -> Product13/2
  Product13/1 -> Product2/2, Product3/1
  Divide/1 -> Subsystem/1(in), Unit Delay/1  "did/dt"
  Sum3/1 -> Divide/2
  Product9/1 -> Sum4/3
  reset/1 -> Subsystem/2(reset), Subsystem1/2(reset)
  u_d/1 -> Sum3/1
  R1/1 -> [R1]
  Subsystem/1(outt) -> I_d/1, [id], Product4/2
  Subsystem1/1(outt) -> [iq], I_q/1, Product9/1  "i_q"
  Product3/1 -> Sum3/4
  Product4/1 -> Sum3/2
  Product2/1 -> Sum4/2  "psi_d*omega_ell"
  Unit Delay/1 -> Product11/1
  Unit Delay1/1 -> Product12/2
  Lqd_approx/1(Lqd) -> [Lqd]  "Lqd"
  Ldq_approx/1(Ldq) -> [Ldq]  "Ldq"
  omega_mech/1 -> Product13/1
  fitting_parameter/1 -> [fitting_para]
  Lqq_approx/1(Lqq) -> Switch8/2, Switch8/1
  Ldd_approx/1(Ldd) -> Switch/2, Switch/1
  Product12/1 -> Sum3/3
  Product11/1 -> Sum4/1
  psiq_approx/1(psiq) -> psi_q/1, [psiq]  "psi_q"
  [fitting_para] -> Lqq_approx/3(FittingParameters)
  [fitting_para] -> Lqd_approx/3(FittingParameters)
  psiq_approx/2(psiq_cross_s1) -> [psiq_cross_s1]
  psid_approx/2(psid_cross_s1) -> [psid_cross_s1]
  psiq_approx/3(psid_cross_s1_integrated) -> [psid_cross_s1_integrated]
  psid_approx/3(psiq_cross_s1_integrated) -> [psiq_cross_s1_integrated]
  Switch8/1 -> [Lqq]
  Switch/1 -> [Ldd]
  Constant1/1 -> Switch8/3
  Constant2/1 -> Switch/3
  [fitting_para] -> Ldd_approx/3(FittingParameters)
  [Lqq] -> Divide1/2
  [iq] -> Lqq_approx/2(Iq)
  [id] -> Ldd_approx/2(Id)
  [Ldd] -> Divide/1
  [psid_cross_s1_integrated] -> Lqq_approx/1(psid_cross_s1_integrated)
  [psiq_cross_s1_integrated] -> Ldd_approx/1(psiq_cross_s1_integrated)
  [psiq_cross_s1] -> Lqd_approx/2(psiq_cross_s1)
  [psiq_cross_s1] -> Ldq_approx/2(psiq_cross_s1)
  [psiq] -> Product3/2
  [iq] -> psiq_approx/2(Iq)
  [id] -> psiq_approx/1(Id)
  [fitting_para] -> psiq_approx/3(FittingParameters)
  [id] -> psid_approx/1(Id)
  [iq] -> psid_approx/2(Iq)
  [fitting_para] -> psid_approx/3(FittingParameters)
  [psid_cross_s1] -> Lqd_approx/1(psid_cross_s1)
  [psid_cross_s1] -> Ldq_approx/1(psid_cross_s1)
  psid_approx/1(psid) -> psi_d/1, [psid]  "psi_d"
  [psid] -> Product2/1
  [fitting_para] -> Ldq_approx/3(FittingParameters)
  [Ldq] -> Product12/1
  [Lqd] -> Product11/2
  [R1] -> Product4/1
  [R1] -> Product9/2

== system uz_pmsm_model_nonlinear/uz_pmsm_model_nonlinear/torque_calculation ==
  I_d : Inport
  psi_d : Inport  Port=2
  psi_q : Inport  Port=3
  polepairs : Inport  Port=4
  I_q : Inport  Port=5
  Factor : Gain  Gain=(3/2)  OutDataTypeStr=Inherit: Same as input
  Product2 : Product  OutDataTypeStr=Inherit: Same as first input
  Product3 : Product  OutDataTypeStr=Inherit: Same as first input
  Product9 : Product  OutDataTypeStr=Inherit: Same as first input
  Sum3 : Sum  Inputs=-|+  OutDataTypeStr=Inherit: Same as first input
  M_Mi : Outport
  wires:
  Sum3/1 -> Factor/1
  Product3/1 -> Sum3/2
  Product2/1 -> Sum3/1
  psi_q/1 -> Product2/2
  psi_d/1 -> Product3/1
  I_d/1 -> Product2/1
  I_q/1 -> Product3/2
  Product9/1 -> M_Mi/1  "M_Mi"
  polepairs/1 -> Product9/2
  Factor/1 -> Product9/1  "M_Mi"

== system uz_pmsm_model_nonlinear/uz_pmsm_model_nonlinear/mechanical_system/integrator1 ==
  reset : Inport
  in : Inport  Port=2
  Delay1 : Delay  DelayLength=1  ExternalReset=Level
      settings: InputPortMap=u0,r5
  Gain : Gain  Gain=ts  OutDataTypeStr=Inherit: Same as input
  Sum3 : Sum  Inputs=|++  OutDataTypeStr=Inherit: Same as first input  LockScale=on
  outt : Outport
  wires:
  in/1 -> Gain/1
  Gain/1 -> Sum3/1
  reset/1 -> Delay1/2
  Sum3/1 -> Delay1/1
  Delay1/1 -> Sum3/2, outt/1

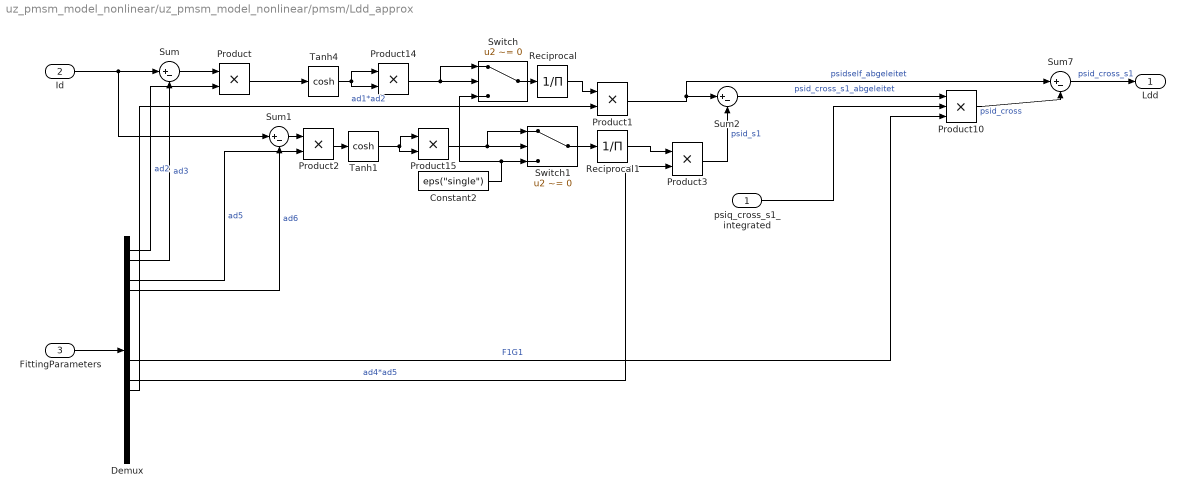
== system uz_pmsm_model_nonlinear/uz_pmsm_model_nonlinear/pmsm/Ldd_approx ==
  psiq_cross_s1_integrated : Inport
  Id : Inport  Port=2
  FittingParameters : Inport  Port=3
  Constant2 : Constant  Value="eps(\"single\")"  OutDataTypeStr=single  SampleTime=ts
  Demux : Demux  Outputs=23
  Product{,1..3} (4 alike) : Product  OutDataTypeStr=single
  Product10 : Product  Inputs=3  OutDataTypeStr=single
  Product14 : Product
  Product15 : Product
  Reciprocal : Product  Inputs=/  RndMeth=Zero  SaturateOnIntegerOverflow=on
  Reciprocal1 : Product  Inputs=/  RndMeth=Zero  SaturateOnIntegerOverflow=on
  Sum : Sum  Inputs=|+-  OutDataTypeStr=single
  Sum1 : Sum  Inputs=|+-  OutDataTypeStr=single
  Sum2 : Sum  Inputs=|+-
  Sum7 : Sum  Inputs=|+-
  Switch : Switch  Criteria=u2 ~= 0  Threshold="eps(\"single\")"  SaturateOnIntegerOverflow=off  InputSameDT=off
  Switch1 : Switch  Criteria=u2 ~= 0  Threshold="eps(\"single\")"  SaturateOnIntegerOverflow=off  InputSameDT=off
  Tanh1 : Trigonometry  Operator=cosh
  Tanh4 : Trigonometry  Operator=cosh
  Ldd : Outport
  wires:
  FittingParameters/1 -> Demux/1
  Demux/3 -> Sum/2  "ad3"
  Sum/1 -> Product/1
  Demux/2 -> Product/2  "ad2"
  Product1/1 -> Sum7/1, Sum2/1  "psidself_abgeleitet"
  Sum1/1 -> Product2/1
  Demux/5 -> Product2/2  "ad5"
  Demux/6 -> Sum1/2  "ad6"
  Id/1 -> Sum1/1, Sum/1
  Product3/1 -> Sum2/2  "psid_s1"
  Sum2/1 -> Product10/1  "psid_cross_s1_abgeleitet"
  Product10/1 -> Sum7/2  "psid_cross"
  Sum7/1 -> Ldd/1  "psid_cross_s1"
  Demux/13 -> Product10/3  "F1G1"
  Tanh4/1 -> Product14/1, Product14/2
  Tanh1/1 -> Product15/1, Product15/2
  Reciprocal1/1 -> Product3/1
  Product/1 -> Tanh4/1
  Product2/1 -> Tanh1/1
  psiq_cross_s1_integrated/1 -> Product10/2
  Reciprocal/1 -> Product1/1
  Demux/15 -> Product3/2  "ad4*ad5"
  Demux/16 -> Product1/2  "ad1*ad2"
  Product14/1 -> Switch/1, Switch/2
  Constant2/1 -> Switch/3, Switch1/3
  Switch/1 -> Reciprocal/1
  Product15/1 -> Switch1/1, Switch1/2
  Switch1/1 -> Reciprocal1/1

== system uz_pmsm_model_nonlinear/uz_pmsm_model_nonlinear/pmsm/Ldq_approx ==
  psid_cross_s1 : Inport
  psiq_cross_s1 : Inport  Port=2
  FittingParameters : Inport  Port=3
  Gain : Gain  Gain=-1
  Product20 : Product  Inputs=3
  Selector : Selector  InputPortWidth=23  IndexOptions=Index vector (dialog)  Indices=[13]  OutputSizes=1
  Ldq : Outport
  wires:
  Product20/1 -> Gain/1
  psid_cross_s1/1 -> Product20/1
  Gain/1 -> Ldq/1
  psiq_cross_s1/1 -> Product20/2
  FittingParameters/1 -> Selector/1
  Selector/1 -> Product20/3

== system uz_pmsm_model_nonlinear/uz_pmsm_model_nonlinear/pmsm/Lqd_approx ==
  psid_cross_s1 : Inport
  psiq_cross_s1 : Inport  Port=2
  FittingParameters : Inport  Port=3
  Gain : Gain  Gain=-1
  Product20 : Product  Inputs=3
  Selector : Selector  InputPortWidth=23  IndexOptions=Index vector (dialog)  Indices=[14]  OutputSizes=1
  Lqd : Outport
  wires:
  FittingParameters/1 -> Selector/1
  Product20/1 -> Gain/1
  psid_cross_s1/1 -> Product20/1
  Gain/1 -> Lqd/1
  psiq_cross_s1/1 -> Product20/2
  Selector/1 -> Product20/3

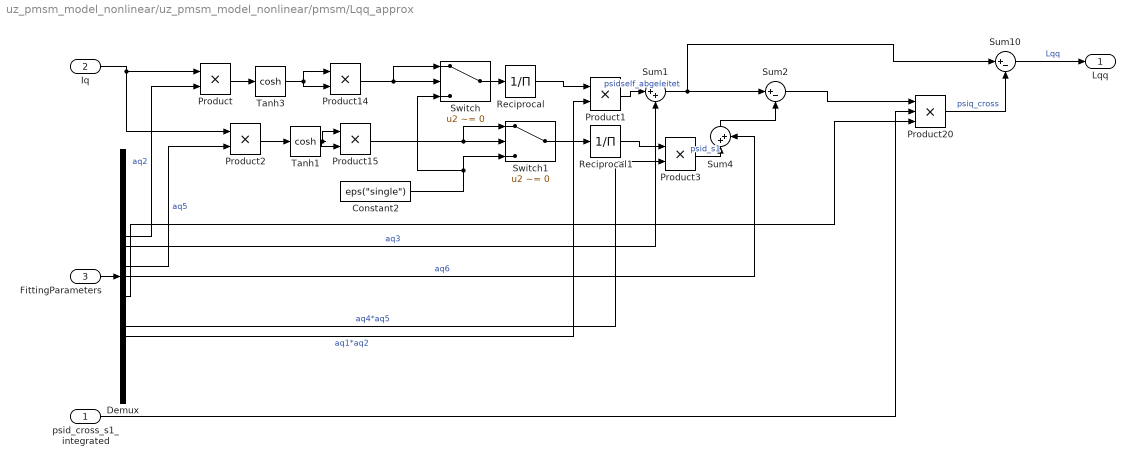
== system uz_pmsm_model_nonlinear/uz_pmsm_model_nonlinear/pmsm/Lqq_approx ==
  psid_cross_s1_integrated : Inport
  Iq : Inport  Port=2
  FittingParameters : Inport  Port=3
  Constant2 : Constant  Value="eps(\"single\")"  OutDataTypeStr=single  SampleTime=ts
  Demux : Demux  Outputs=23
  Product : Product  OutDataTypeStr=Inherit: Same as first input
  Product{1,3,14..15} (4 alike) : Product
  Product2 : Product  OutDataTypeStr=Inherit: Same as first input
  Product20 : Product  Inputs=3
  Reciprocal : Product  Inputs=/  RndMeth=Zero  SaturateOnIntegerOverflow=on
  Reciprocal1 : Product  Inputs=/  RndMeth=Zero  SaturateOnIntegerOverflow=on
  Sum1 : Sum  Inputs=|++
  Sum10 : Sum  Inputs=|+-
  Sum2 : Sum  Inputs=|+-
  Sum4 : Sum  Inputs=|++
  Switch : Switch  Criteria=u2 ~= 0  Threshold="eps(\"single\")"  SaturateOnIntegerOverflow=off  InputSameDT=off
  Switch1 : Switch  Criteria=u2 ~= 0  Threshold="eps(\"single\")"  SaturateOnIntegerOverflow=off  InputSameDT=off
  Tanh1 : Trigonometry  Operator=cosh
  Tanh3 : Trigonometry  Operator=cosh
  Lqq : Outport
  wires:
  FittingParameters/1 -> Demux/1
  Demux/12 -> Sum4/2  "aq6"
  Product20/1 -> Sum10/2  "psiq_cross"
  Sum10/1 -> Lqq/1  "Lqq"
  Demux/14 -> Product20/3
  Demux/9 -> Sum1/2  "aq3"
  Tanh3/1 -> Product14/1, Product14/2
  Tanh1/1 -> Product15/2, Product15/1
  Sum2/1 -> Product20/1
  Reciprocal/1 -> Product1/1
  Reciprocal1/1 -> Product3/1
  Demux/8 -> Product/2  "aq2"
  Iq/1 -> Product2/1, Product/1
  Demux/11 -> Product2/2  "aq5"
  Product1/1 -> Sum1/1  "psidself_abgeleitet"
  Sum1/1 -> Sum10/1, Sum2/1
  Sum4/1 -> Sum2/2
  Product3/1 -> Sum4/1  "psid_s1"
  Product2/1 -> Tanh1/1
  Product/1 -> Tanh3/1
  psid_cross_s1_integrated/1 -> Product20/2
  Demux/18 -> Product1/2  "aq1*aq2"
  Demux/17 -> Product3/2  "aq4*aq5"
  Product14/1 -> Switch/2, Switch/1
  Constant2/1 -> Switch/3, Switch1/3
  Switch/1 -> Reciprocal/1
  Product15/1 -> Switch1/2, Switch1/1
  Switch1/1 -> Reciprocal1/1

== system uz_pmsm_model_nonlinear/uz_pmsm_model_nonlinear/pmsm/Subsystem ==
  in : Inport
  reset : Inport  Port=2
  Delay1 : Delay  DelayLength=1  ExternalReset=Level
      settings: InputPortMap=u0,r5
  Gain7 : Gain  Gain=ts  OutDataTypeStr=Inherit: Same as input
  Sum5 : Sum  Inputs=|++  OutDataTypeStr=Inherit: Same as first input
  outt : Outport
  wires:
  in/1 -> Gain7/1
  reset/1 -> Delay1/2
  Delay1/1 -> outt/1, Sum5/2
  Sum5/1 -> Delay1/1
  Gain7/1 -> Sum5/1  "u_d"

== system uz_pmsm_model_nonlinear/uz_pmsm_model_nonlinear/pmsm/Subsystem1 ==
  in : Inport
  reset : Inport  Port=2
  Delay1 : Delay  DelayLength=1  ExternalReset=Level
      settings: InputPortMap=u0,r5
  Gain7 : Gain  Gain=ts
  Sum5 : Sum  Inputs=|++  OutDataTypeStr=Inherit: Same as first input
  outt : Outport
  wires:
  in/1 -> Gain7/1
  reset/1 -> Delay1/2
  Delay1/1 -> outt/1, Sum5/2
  Sum5/1 -> Delay1/1
  Gain7/1 -> Sum5/1  "u_d"

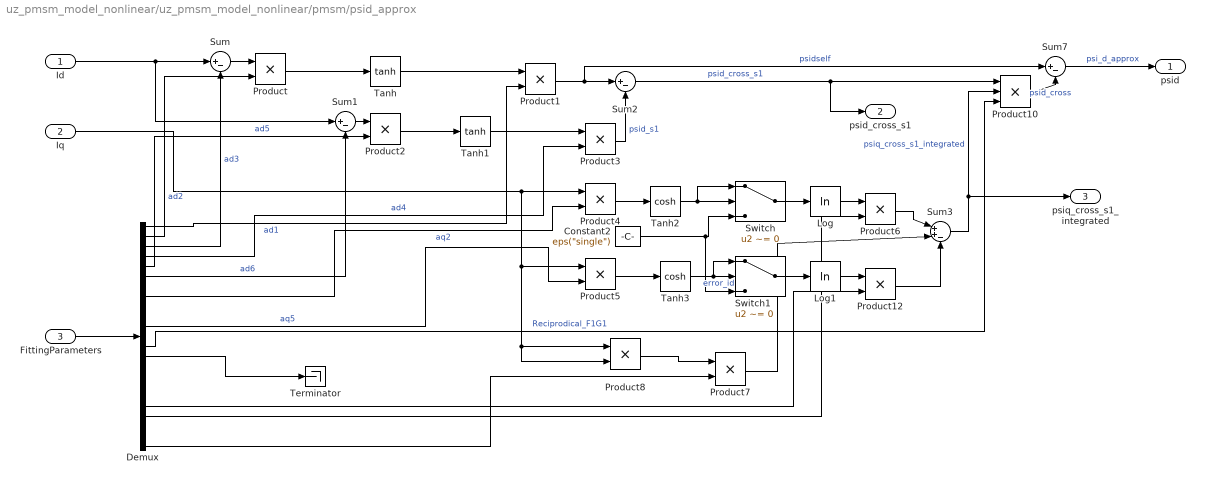
== system uz_pmsm_model_nonlinear/uz_pmsm_model_nonlinear/pmsm/psid_approx ==
  Id : Inport
  Iq : Inport  Port=2
  FittingParameters : Inport  Port=3
  Constant2 : Constant  Value="eps(\"single\")"  OutDataTypeStr=single  SampleTime=ts
  Demux : Demux  Outputs=23
  Log : Math  Operator=log  SignedPower=on
  Log1 : Math  Operator=log  SignedPower=on
  Product{,2,4..5,8} (5 alike) : Product  OutDataTypeStr=Inherit: Same as first input
  Product{1,3,6..7,12} (5 alike) : Product
  Product10 : Product  Inputs=3
  Sum{,1..2,7} (4 alike) : Sum  Inputs=|+-
  Sum3 : Sum  Inputs=|++-
  Switch : Switch  Criteria=u2 ~= 0  Threshold="eps(\"single\")"  SaturateOnIntegerOverflow=off  InputSameDT=off
  Switch1 : Switch  Criteria=u2 ~= 0  Threshold="eps(\"single\")"  SaturateOnIntegerOverflow=off  InputSameDT=off
  Tanh : Trigonometry  Operator=tanh
  Tanh1 : Trigonometry  Operator=tanh
  Tanh2 : Trigonometry  Operator=cosh
  Tanh3 : Trigonometry  Operator=cosh
  Terminator : Terminator
  psid : Outport
  psid_cross_s1 : Outport  Port=2
  psiq_cross_s1_integrated : Outport  Port=3
  wires:
  FittingParameters/1 -> Demux/1
  Demux/1 -> Product1/2  "ad1"
  Demux/3 -> Sum/2  "ad3"
  Sum/1 -> Product/1
  Demux/2 -> Product/2  "ad2"
  Product1/1 -> Sum7/1, Sum2/1  "psidself"
  Demux/4 -> Product3/2  "ad4"
  Sum1/1 -> Product2/1
  Demux/5 -> Product2/2  "ad5"
  Demux/6 -> Sum1/2  "ad6"
  Id/1 -> Sum1/1, Sum/1
  Product3/1 -> Sum2/2  "psid_s1"
  Iq/1 -> Product8/2, Product8/1, Product5/1, Product4/1
  Sum2/1 -> psid_cross_s1/1, Product10/1  "psid_cross_s1"
  Product8/1 -> Product7/1
  Product7/1 -> Sum3/2
  Demux/20 -> Product6/2
  Product6/1 -> Sum3/1
  Demux/19 -> Product12/2
  Product12/1 -> Sum3/3
  Sum3/1 -> Product10/2, psiq_cross_s1_integrated/1  "psiq_cross_s1_integrated"
  Demux/11 -> Product5/2  "aq5"
  Demux/8 -> Product4/2  "aq2"
  Product10/1 -> Sum7/2  "psid_cross"
  Sum7/1 -> psid/1  "psi_d_approx"
  Demux/14 -> Terminator/1
  Demux/13 -> Product10/3  "Reciprodical_F1G1"
  Log/1 -> Product6/1
  Log1/1 -> Product12/1
  Tanh/1 -> Product1/1
  Tanh1/1 -> Product3/1
  Product/1 -> Tanh/1
  Product2/1 -> Tanh1/1
  Product4/1 -> Tanh2/1
  Product5/1 -> Tanh3/1
  Demux/23 -> Product7/2
  Tanh2/1 -> Switch/1, Switch/2
  Switch/1 -> Log/1
  Tanh3/1 -> Switch1/2, Switch1/1  "error_id"
  Constant2/1 -> Switch1/3, Switch/3
  Switch1/1 -> Log1/1

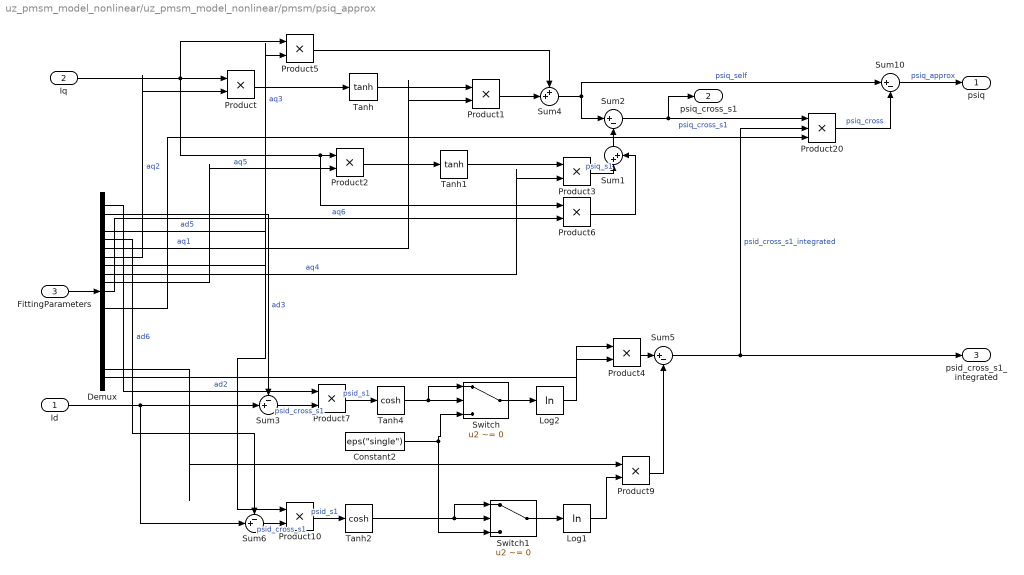
== system uz_pmsm_model_nonlinear/uz_pmsm_model_nonlinear/pmsm/psiq_approx ==
  Id : Inport
  Iq : Inport  Port=2
  FittingParameters : Inport  Port=3
  Constant2 : Constant  Value="eps(\"single\")"  OutDataTypeStr=single  SampleTime=ts
  Demux : Demux  Outputs=23
  Log1 : Math  Operator=log  SignedPower=on
  Log2 : Math  Operator=log  SignedPower=on
  Product{,2,7,10} (4 alike) : Product  OutDataTypeStr=Inherit: Same as first input
  Product{1,3..6,9} (6 alike) : Product
  Product20 : Product  Inputs=3
  Sum1 : Sum  Inputs=|++
  Sum10 : Sum  Inputs=|+-
  Sum2 : Sum  Inputs=|+-
  Sum3 : Sum  Inputs=-+|
  Sum4 : Sum  Inputs=++|
  Sum5 : Sum  Inputs=|+-
  Sum6 : Sum  Inputs=-+|
  Switch : Switch  Criteria=u2 ~= 0  Threshold="eps(\"single\")"  SaturateOnIntegerOverflow=off  InputSameDT=off
  Switch1 : Switch  Criteria=u2 ~= 0  Threshold="eps(\"single\")"  SaturateOnIntegerOverflow=off  InputSameDT=off
  Tanh : Trigonometry  Operator=tanh
  Tanh1 : Trigonometry  Operator=tanh
  Tanh2 : Trigonometry  Operator=cosh
  Tanh4 : Trigonometry  Operator=cosh
  psiq : Outport
  psiq_cross_s1 : Outport  Port=2
  psid_cross_s1_integrated : Outport  Port=3
  wires:
  FittingParameters/1 -> Demux/1
  Sum2/1 -> Product20/1, psiq_cross_s1/1  "psiq_cross_s1"
  Demux/10 -> Product3/2  "aq4"
  Demux/12 -> Product6/2  "aq6"
  Demux/8 -> Product/2  "aq2"
  Demux/11 -> Product2/2  "aq5"
  Demux/7 -> Product1/2  "aq1"
  Iq/1 -> Product2/1, Product6/1, Product/1, Product5/1
  Demux/9 -> Product5/2  "aq3"
  Demux/22 -> Product4/1
  Product1/1 -> Sum4/2
  Product5/1 -> Sum4/1
  Sum4/1 -> Sum10/1, Sum2/1  "psiq_self"
  Sum1/1 -> Sum2/2
  Product3/1 -> Sum1/1  "psiq_s1"
  Product6/1 -> Sum1/2
  Sum3/1 -> Product7/2  "psid_cross_s1"
  Product7/1 -> Tanh4/1  "psid_s1"
  Product4/1 -> Sum5/1
  Product9/1 -> Sum5/2
  Product10/1 -> Tanh2/1  "psid_s1"
  Demux/21 -> Product9/1
  Sum6/1 -> Product10/2  "psid_cross_s1"
  Demux/3 -> Sum3/1  "ad3"
  Demux/2 -> Product7/1  "ad2"
  Demux/5 -> Product10/1  "ad5"
  Demux/6 -> Sum6/1  "ad6"
  Id/1 -> Sum6/2, Sum3/2
  Sum5/1 -> psid_cross_s1_integrated/1, Product20/2  "psid_cross_s1_integrated"
  Product20/1 -> Sum10/2  "psiq_cross"
  Sum10/1 -> psiq/1  "psiq_approx"
  Demux/14 -> Product20/3
  Log1/1 -> Product9/2
  Log2/1 -> Product4/2
  Tanh1/1 -> Product3/1
  Tanh/1 -> Product1/1
  Product2/1 -> Tanh1/1
  Product/1 -> Tanh/1
  Tanh4/1 -> Switch/1, Switch/2
  Switch/1 -> Log2/1
  Constant2/1 -> Switch/3, Switch1/3
  Tanh2/1 -> Switch1/1, Switch1/2
  Switch1/1 -> Log1/1
